simulink model "final_heart_sym3_2_Level_hdl"  (R2021a)
settings: Solver=VariableStepAuto  StartTime=0.0  StopTime=10.0  RelTol=1e-3
undefined symbols (not defined in the file or in its folder): lambda2
(part 1 of 2)
settings Model: Creator=Acer  LastModifiedBy=Acer

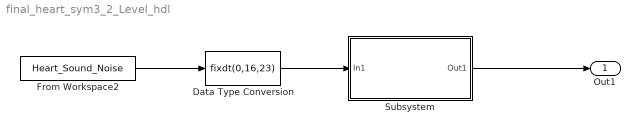
== system final_heart_sym3_2_Level_hdl ==
  Data Type Conversion : DataTypeConversion  OutDataTypeStr=fixdt(0,16,23)
  From Workspace2 : FromWorkspace  VariableName=Heart_Sound_Noise  OutDataTypeStr=double  SampleTime=1/44100
  Subsystem : Subsystem
  Out1 : Outport  OutDataTypeStr=fixdt(1,16,29)  SampleTime=1/44100
  wires:
  Subsystem/1(Out1) -> Out1/1
  From Workspace2/1 -> Data Type Conversion/1
  Data Type Conversion/1 -> Subsystem/1(In1)

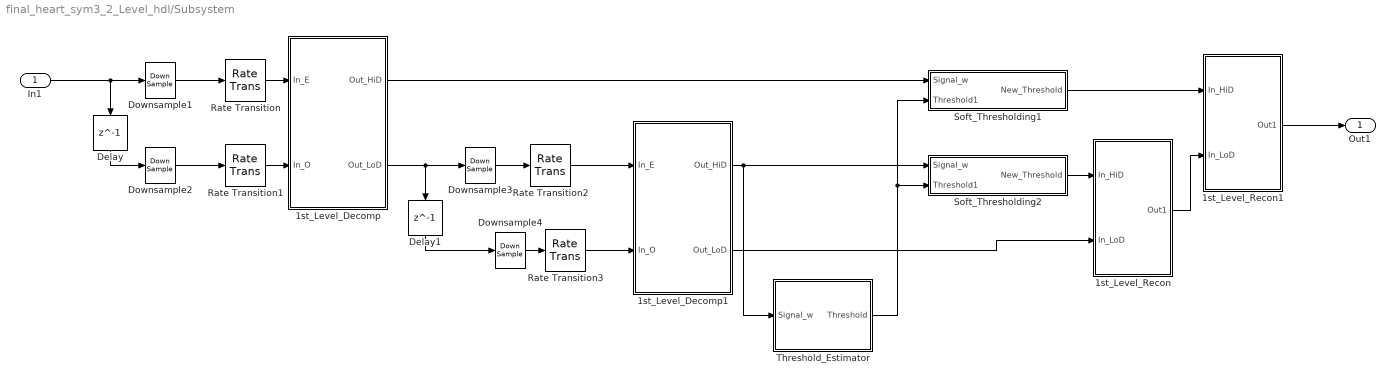
== system final_heart_sym3_2_Level_hdl/Subsystem ==
  In1 : Inport  OutDataTypeStr=fixdt(0,16,23)
  1st_Level_Decomp : Subsystem
  1st_Level_Decomp1 : Subsystem
  1st_Level_Recon : Subsystem
  1st_Level_Recon1 : Subsystem
  Delay : Delay  DelayLength=1  SampleTime=1/44100
  Delay1 : Delay  DelayLength=1  SampleTime=1/44100
  Downsample{1..4} (4 alike) : DownSample  N=30  RateOptions=Allow multirate processing
  Rate Transition{,1..3} (4 alike) : RateTransition
  Soft_Thresholding1 : Subsystem
  Soft_Thresholding2 : Subsystem
  Threshold_Estimator : Subsystem
  Out1 : Outport  OutDataTypeStr=fixdt(1,16,29)  SampleTime=1/44100
  wires:
  Rate Transition3/1 -> 1st_Level_Decomp1/2(In_O)
  Rate Transition1/1 -> 1st_Level_Decomp/2(In_O)
  1st_Level_Decomp1/1(Out_HiD) -> Threshold_Estimator/1(Signal_w), Soft_Thresholding2/1(Signal_w)
  Delay/1 -> Downsample2/1
  Soft_Thresholding1/1(New_Threshold) -> 1st_Level_Recon1/1(In_HiD)
  Downsample2/1 -> Rate Transition1/1
  1st_Level_Decomp/1(Out_HiD) -> Soft_Thresholding1/1(Signal_w)
  Delay1/1 -> Downsample4/1
  Downsample4/1 -> Rate Transition3/1
  1st_Level_Recon1/1(Out1) -> Out1/1
  Rate Transition2/1 -> 1st_Level_Decomp1/1(In_E)
  In1/1 -> Delay/1, Downsample1/1
  1st_Level_Decomp/2(Out_LoD) -> Downsample3/1, Delay1/1
  Soft_Thresholding2/1(New_Threshold) -> 1st_Level_Recon/1(In_HiD)
  Threshold_Estimator/1(Threshold) -> Soft_Thresholding2/2(Threshold1), Soft_Thresholding1/2(Threshold1)
  Downsample1/1 -> Rate Transition/1
  1st_Level_Recon/1(Out1) -> 1st_Level_Recon1/2(In_LoD)
  Rate Transition/1 -> 1st_Level_Decomp/1(In_E)
  Downsample3/1 -> Rate Transition2/1
  1st_Level_Decomp1/2(Out_LoD) -> 1st_Level_Recon/2(In_LoD)

== system final_heart_sym3_2_Level_hdl/Subsystem/1st_Level_Decomp ==
  In_E : Inport  OutDataTypeStr=fixdt(0,16,23)  SampleTime=1/44100
  In_O : Inport  Port=2  OutDataTypeStr=fixdt(0,16,23)  SampleTime=1/44100
  Add : Sum  AccumDataTypeStr=fixdt(1,16,23)  OutDataTypeStr=fixdt(1,16,24)
  Add1 : Sum  AccumDataTypeStr=fixdt(1,16,22)  OutDataTypeStr=fixdt(1,16,22)
  Delay1 : Delay  DelayLength=1  SampleTime=1/44100
  Delay2 : Delay  DelayLength=1  SampleTime=1/44100
  Gain : Gain  Gain=1/(0.877989329+0.977128821)  ParamDataTypeStr=fixdt(0,16,16)  OutDataTypeStr=fixdt(1,16,24)
  Gain1 : Gain  Gain=1/(0.877989329+0.977128821)  ParamDataTypeStr=fixdt(0,16,16)  OutDataTypeStr=fixdt(1,16,23)
  HiD_Even : Subsystem
  HiD_Odd : Subsystem
  LoD_Even : Subsystem
  LoD_Odd : Subsystem
  Out_HiD : Outport  OutDataTypeStr=fixdt(1,16,24)  SampleTime=1/44100  VectorParamsAs1DForOutWhenUnconnected=off
  Out_LoD : Outport  Port=2  OutDataTypeStr=fixdt(1,16,23)  SampleTime=1/44100  VectorParamsAs1DForOutWhenUnconnected=off
  wires:
  HiD_Odd/1(Out_HiD_o) -> Add/2
  HiD_Even/1(Out_HiD_e) -> Add/1
  LoD_Odd/1(Out_LoD_o) -> Add1/2
  LoD_Even/1(Out_LoD_e) -> Add1/1
  In_E/1 -> LoD_Even/1(In_LoD_e), HiD_Even/1(In_HiD_e)
  In_O/1 -> LoD_Odd/1(In_LoD_o), HiD_Odd/1(In_HiD_o)
  Gain/1 -> Delay1/1
  Delay1/1 -> Out_HiD/1
  Delay2/1 -> Out_LoD/1
  Add/1 -> Gain/1
  Add1/1 -> Gain1/1
  Gain1/1 -> Delay2/1

== system final_heart_sym3_2_Level_hdl/Subsystem/1st_Level_Decomp1 ==
  In_E : Inport  OutDataTypeStr=fixdt(1,16,4)  SampleTime=1/44100
  In_O : Inport  Port=2  OutDataTypeStr=fixdt(1,16,4)  SampleTime=1/44100
  Add : Sum  AccumDataTypeStr=fixdt(1,16,4)  OutDataTypeStr=fixdt(1,16,4)
  Add1 : Sum  AccumDataTypeStr=fixdt(1,16,4)  OutDataTypeStr=fixdt(1,16,4)
  Delay1 : Delay  DelayLength=1  SampleTime=1/44100
  Delay2 : Delay  DelayLength=1  SampleTime=1/44100
  Gain : Gain  Gain=1/(0.877989329+0.977128821)  ParamDataTypeStr=fixdt(0,16,16)  OutDataTypeStr=fixdt(1,16,4)
  Gain1 : Gain  Gain=1/(0.877989329+0.977128821)  ParamDataTypeStr=fixdt(0,16,16)  OutDataTypeStr=fixdt(1,16,4)
  HiD_Even : Subsystem
  HiD_Odd : Subsystem
  LoD_Even : Subsystem
  LoD_Odd : Subsystem
  Out_HiD : Outport  OutDataTypeStr=fixdt(1,16,4)  SampleTime=1/44100  VectorParamsAs1DForOutWhenUnconnected=off
  Out_LoD : Outport  Port=2  OutDataTypeStr=fixdt(1,16,4)  SampleTime=1/44100  VectorParamsAs1DForOutWhenUnconnected=off
  wires:
  HiD_Odd/1(Out_HiD_o) -> Add/2
  HiD_Even/1(Out_HiD_e) -> Add/1
  LoD_Odd/1(Out_LoD_o) -> Add1/2
  LoD_Even/1(Out_LoD_e) -> Add1/1
  In_E/1 -> LoD_Even/1(In_LoD_e), HiD_Even/1(In_HiD_e)
  In_O/1 -> LoD_Odd/1(In_LoD_o), HiD_Odd/1(In_HiD_o)
  Gain/1 -> Delay1/1
  Delay1/1 -> Out_HiD/1
  Delay2/1 -> Out_LoD/1
  Add/1 -> Gain/1
  Add1/1 -> Gain1/1
  Gain1/1 -> Delay2/1

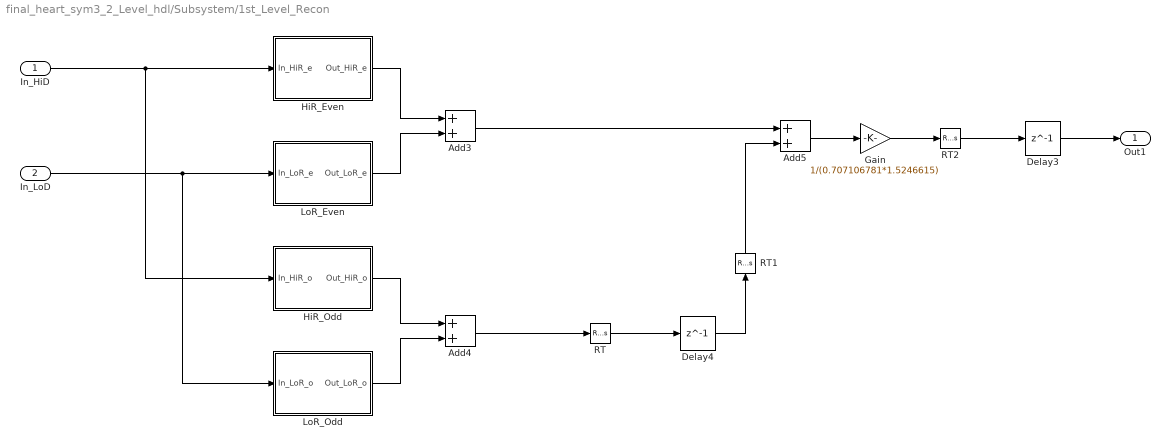
== system final_heart_sym3_2_Level_hdl/Subsystem/1st_Level_Recon ==
  In_HiD : Inport  OutDataTypeStr=fixdt(1,16,4)  SampleTime=1/44100
  In_LoD : Inport  Port=2  OutDataTypeStr=fixdt(1,16,4)  SampleTime=1/44100
  Add3 : Sum  AccumDataTypeStr=fixdt(1,16,4)  OutDataTypeStr=fixdt(1,16,4)
  Add4 : Sum  AccumDataTypeStr=fixdt(1,16,4)  OutDataTypeStr=fixdt(1,16,4)
  Add5 : Sum  AccumDataTypeStr=fixdt(1,16,4)  OutDataTypeStr=fixdt(1,16,4)
  Delay3 : Delay  DelayLength=1  SampleTime=1/44100
  Delay4 : Delay  DelayLength=1  SampleTime=1/44100
  Gain : Gain  Gain=1/(0.707106781*1.5246615)  ParamDataTypeStr=fixdt(0,16,16)  OutDataTypeStr=fixdt(1,16,4)
  HiR_Even : Subsystem
  HiR_Odd : Subsystem
  LoR_Even : Subsystem
  LoR_Odd : Subsystem
  RT : RateTransition
  RT1 : RateTransition
  RT2 : RateTransition
  Out1 : Outport  OutDataTypeStr=fixdt(1,16,4)  SampleTime=1/44100
  wires:
  In_HiD/1 -> HiR_Odd/1(In_HiR_o), HiR_Even/1(In_HiR_e)
  HiR_Even/1(Out_HiR_e) -> Add3/1
  In_LoD/1 -> LoR_Odd/1(In_LoR_o), LoR_Even/1(In_LoR_e)
  LoR_Even/1(Out_LoR_e) -> Add3/2
  HiR_Odd/1(Out_HiR_o) -> Add4/1
  LoR_Odd/1(Out_LoR_o) -> Add4/2
  RT/1 -> Delay4/1
  Delay3/1 -> Out1/1
  RT1/1 -> Add5/2
  RT2/1 -> Delay3/1
  Delay4/1 -> RT1/1
  Add5/1 -> Gain/1
  Gain/1 -> RT2/1
  Add3/1 -> Add5/1
  Add4/1 -> RT/1

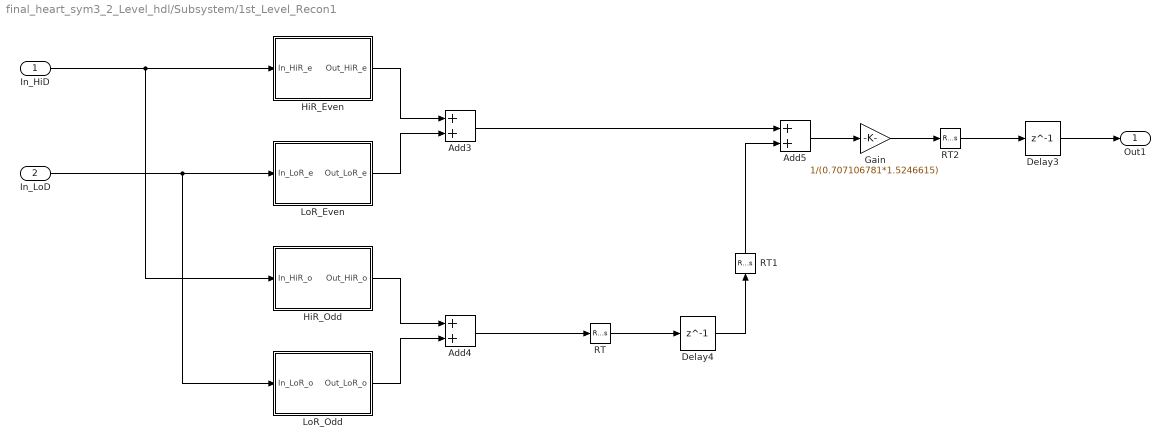
== system final_heart_sym3_2_Level_hdl/Subsystem/1st_Level_Recon1 ==
  In_HiD : Inport  OutDataTypeStr=fixdt(1,16,28)  SampleTime=1/44100
  In_LoD : Inport  Port=2  OutDataTypeStr=fixdt(1,16,4)  SampleTime=1/44100
  Add3 : Sum  AccumDataTypeStr=fixdt(1,16,28)  OutDataTypeStr=fixdt(1,16,28)
  Add4 : Sum  AccumDataTypeStr=fixdt(1,16,28)  OutDataTypeStr=fixdt(1,16,28)
  Add5 : Sum  AccumDataTypeStr=fixdt(1,16,28)  OutDataTypeStr=fixdt(1,16,29)
  Delay3 : Delay  DelayLength=1  SampleTime=1/44100
  Delay4 : Delay  DelayLength=1  SampleTime=1/44100
  Gain : Gain  Gain=1/(0.707106781*1.5246615)  ParamDataTypeStr=fixdt(0,16,16)  OutDataTypeStr=fixdt(1,16,29)
  HiR_Even : Subsystem
  HiR_Odd : Subsystem
  LoR_Even : Subsystem
  LoR_Odd : Subsystem
  RT : RateTransition
  RT1 : RateTransition
  RT2 : RateTransition
  Out1 : Outport  OutDataTypeStr=fixdt(1,16,29)  SampleTime=1/44100
  wires:
  In_HiD/1 -> HiR_Odd/1(In_HiR_o), HiR_Even/1(In_HiR_e)
  HiR_Even/1(Out_HiR_e) -> Add3/1
  In_LoD/1 -> LoR_Odd/1(In_LoR_o), LoR_Even/1(In_LoR_e)
  LoR_Even/1(Out_LoR_e) -> Add3/2
  HiR_Odd/1(Out_HiR_o) -> Add4/1
  LoR_Odd/1(Out_LoR_o) -> Add4/2
  RT/1 -> Delay4/1
  Delay3/1 -> Out1/1
  RT1/1 -> Add5/2
  RT2/1 -> Delay3/1
  Delay4/1 -> RT1/1
  Add5/1 -> Gain/1
  Gain/1 -> RT2/1
  Add3/1 -> Add5/1
  Add4/1 -> RT/1

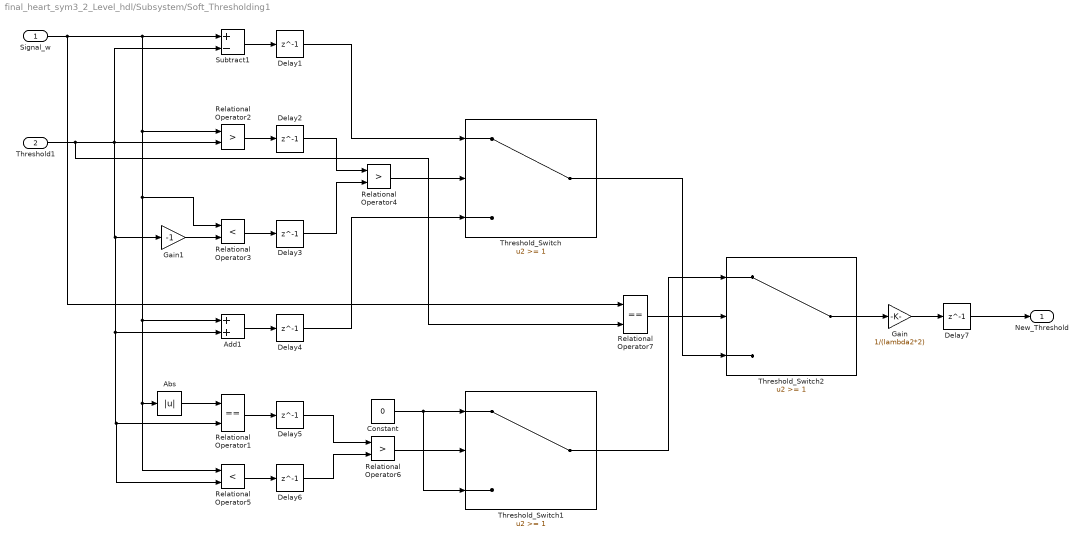
== system final_heart_sym3_2_Level_hdl/Subsystem/Soft_Thresholding1 ==
  Signal_w : Inport  OutDataTypeStr=fixdt(1,16,24)  SampleTime=1/44100
  Threshold1 : Inport  Port=2  OutDataTypeStr=fixdt(1,16,4)  SampleTime=1/44100
  Abs : Abs  OutDataTypeStr=fixdt(0,16,25)
  Add1 : Sum  AccumDataTypeStr=fixdt(1,16,24)  OutDataTypeStr=fixdt(1,16,24)
  Constant : Constant  Value=0  OutDataTypeStr=fixdt(1,16,4)  SampleTime=1/44100
  Delay{1..7} (7 alike) : Delay  DelayLength=1  SampleTime=1/44100
  Gain : Gain  Gain=1/(lambda2*2)  ParamDataTypeStr=fixdt(0,16,19)  OutDataTypeStr=fixdt(1,16,28)
  Gain1 : Gain  Gain=-1  ParamDataTypeStr=fixdt(1,16,15)  OutMin=-1  OutMax=-0.99  OutDataTypeStr=fixdt(1,16,15)
  Relational Operator1 : RelationalOperator  Operator===  OutDataTypeStr=boolean  RndMeth=Simplest
  Relational Operator2 : RelationalOperator  Operator=>  OutDataTypeStr=boolean  RndMeth=Simplest
  Relational Operator3 : RelationalOperator  Operator=<  OutDataTypeStr=boolean  RndMeth=Simplest
  Relational Operator4 : RelationalOperator  Operator=>  OutDataTypeStr=boolean  RndMeth=Simplest
  Relational Operator5 : RelationalOperator  Operator=<  OutDataTypeStr=boolean  RndMeth=Simplest
  Relational Operator6 : RelationalOperator  Operator=>  OutDataTypeStr=boolean  RndMeth=Simplest
  Relational Operator7 : RelationalOperator  Operator===  OutDataTypeStr=boolean  RndMeth=Simplest
  Subtract1 : Sum  Inputs=+-  AccumDataTypeStr=fixdt(1,16,24)  OutDataTypeStr=fixdt(1,16,24)
  Threshold_Switch : Switch  Threshold=1  OutDataTypeStr=fixdt(1,16,24)
  Threshold_Switch1 : Switch  Threshold=1  OutDataTypeStr=fixdt(1,16,4)
  Threshold_Switch2 : Switch  Threshold=1  OutDataTypeStr=fixdt(1,16,24)
  New_Threshold : Outport  OutDataTypeStr=fixdt(1,16,28)  SampleTime=1/44100
  wires:
  Threshold_Switch/1 -> Threshold_Switch2/3
  Relational Operator6/1 -> Threshold_Switch1/2
  Gain1/1 -> Relational Operator3/2
  Delay4/1 -> Threshold_Switch/3
  Add1/1 -> Delay4/1
  Delay2/1 -> Relational Operator4/1
  Delay3/1 -> Relational Operator4/2
  Delay1/1 -> Threshold_Switch/1
  Relational Operator2/1 -> Delay2/1
  Relational Operator3/1 -> Delay3/1
  Relational Operator5/1 -> Delay6/1
  Delay6/1 -> Relational Operator6/2
  Delay5/1 -> Relational Operator6/1
  Threshold1/1 -> Relational Operator2/2, Subtract1/2, Relational Operator5/2, Relational Operator1/2, Add1/2, Gain1/1, Relational Operator7/2
  Abs/1 -> Relational Operator1/1
  Relational Operator4/1 -> Threshold_Switch/2
  Subtract1/1 -> Delay1/1
  Constant/1 -> Threshold_Switch1/3, Threshold_Switch1/1
  Signal_w/1 -> Subtract1/1, Relational Operator2/1, Relational Operator5/1, Abs/1, Add1/1, Relational Operator3/1, Relational Operator7/1
  Relational Operator7/1 -> Threshold_Switch2/2
  Relational Operator1/1 -> Delay5/1
  Threshold_Switch1/1 -> Threshold_Switch2/1
  Delay7/1 -> New_Threshold/1
  Threshold_Switch2/1 -> Gain/1
  Gain/1 -> Delay7/1

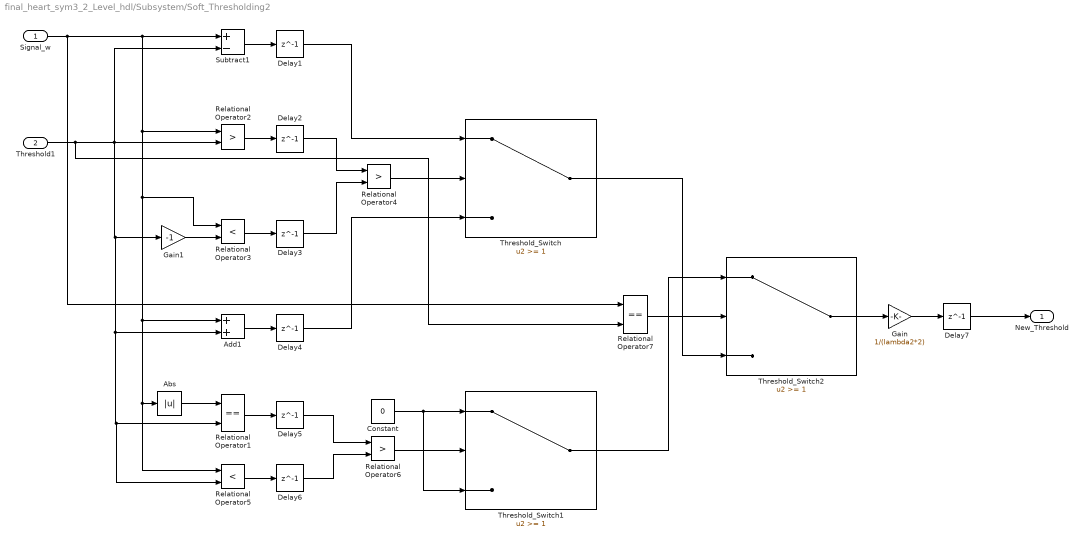
== system final_heart_sym3_2_Level_hdl/Subsystem/Soft_Thresholding2 ==
  Signal_w : Inport  OutDataTypeStr=fixdt(1,16,4)  SampleTime=1/44100
  Threshold1 : Inport  Port=2  OutDataTypeStr=fixdt(1,16,4)  SampleTime=1/44100
  Abs : Abs  OutDataTypeStr=fixdt(1,16,4)
  Add1 : Sum  AccumDataTypeStr=fixdt(1,16,4)  OutDataTypeStr=fixdt(1,16,4)
  Constant : Constant  Value=0  OutDataTypeStr=fixdt(1,16,4)  SampleTime=1/44100
  Delay{1..7} (7 alike) : Delay  DelayLength=1  SampleTime=1/44100
  Gain : Gain  Gain=1/(lambda2*2)  ParamDataTypeStr=fixdt(0,16,19)  OutDataTypeStr=fixdt(1,16,4)
  Gain1 : Gain  Gain=-1  ParamDataTypeStr=fixdt(1,16,15)  OutMin=-1  OutMax=-0.99  OutDataTypeStr=fixdt(1,16,15)
  Relational Operator1 : RelationalOperator  Operator===  OutDataTypeStr=boolean  RndMeth=Simplest
  Relational Operator2 : RelationalOperator  Operator=>  OutDataTypeStr=boolean  RndMeth=Simplest
  Relational Operator3 : RelationalOperator  Operator=<  OutDataTypeStr=boolean  RndMeth=Simplest
  Relational Operator4 : RelationalOperator  Operator=>  OutDataTypeStr=boolean  RndMeth=Simplest
  Relational Operator5 : RelationalOperator  Operator=<  OutDataTypeStr=boolean  RndMeth=Simplest
  Relational Operator6 : RelationalOperator  Operator=>  OutDataTypeStr=boolean  RndMeth=Simplest
  Relational Operator7 : RelationalOperator  Operator===  OutDataTypeStr=boolean  RndMeth=Simplest
  Subtract1 : Sum  Inputs=+-  AccumDataTypeStr=fixdt(1,16,4)  OutDataTypeStr=fixdt(1,16,4)
  Threshold_Switch : Switch  Threshold=1  OutDataTypeStr=fixdt(1,16,4)
  Threshold_Switch1 : Switch  Threshold=1  OutDataTypeStr=fixdt(1,16,4)
  Threshold_Switch2 : Switch  Threshold=1  OutDataTypeStr=fixdt(1,16,4)
  New_Threshold : Outport  OutDataTypeStr=fixdt(1,16,4)  SampleTime=1/44100
  wires:
  Threshold_Switch/1 -> Threshold_Switch2/3
  Relational Operator6/1 -> Threshold_Switch1/2
  Gain1/1 -> Relational Operator3/2
  Delay4/1 -> Threshold_Switch/3
  Add1/1 -> Delay4/1
  Delay2/1 -> Relational Operator4/1
  Delay3/1 -> Relational Operator4/2
  Delay1/1 -> Threshold_Switch/1
  Relational Operator2/1 -> Delay2/1
  Relational Operator3/1 -> Delay3/1
  Relational Operator5/1 -> Delay6/1
  Delay6/1 -> Relational Operator6/2
  Delay5/1 -> Relational Operator6/1
  Threshold1/1 -> Relational Operator2/2, Subtract1/2, Relational Operator5/2, Relational Operator1/2, Add1/2, Gain1/1, Relational Operator7/2
  Abs/1 -> Relational Operator1/1
  Relational Operator4/1 -> Threshold_Switch/2
  Subtract1/1 -> Delay1/1
  Constant/1 -> Threshold_Switch1/3, Threshold_Switch1/1
  Signal_w/1 -> Subtract1/1, Relational Operator2/1, Relational Operator5/1, Abs/1, Add1/1, Relational Operator3/1, Relational Operator7/1
  Relational Operator7/1 -> Threshold_Switch2/2
  Relational Operator1/1 -> Delay5/1
  Threshold_Switch1/1 -> Threshold_Switch2/1
  Delay7/1 -> New_Threshold/1
  Threshold_Switch2/1 -> Gain/1
  Gain/1 -> Delay7/1

== system final_heart_sym3_2_Level_hdl/Subsystem/Threshold_Estimator ==
  Signal_w : Inport  OutDataTypeStr=fixdt(1,16,4)  SampleTime=1/44100
  Absolute_Value1 : Subsystem
  Length : Constant  Value=lambda2  OutDataTypeStr=fixdt(0,16,13)  SampleTime=1/44100
  Median2 : Subsystem
  Multiply : Product  OutDataTypeStr=fixdt(1,16,4)
  Threshold : Outport  OutDataTypeStr=fixdt(1,16,4)  SampleTime=1/44100  VectorParamsAs1DForOutWhenUnconnected=off
  wires:
  Length/1 -> Multiply/2
  Median2/1(Median) -> Multiply/1
  Absolute_Value1/1(Out_Abs) -> Median2/1(Signal_w3)
  Signal_w/1 -> Absolute_Value1/1(Signal_w4)
  Multiply/1 -> Threshold/1

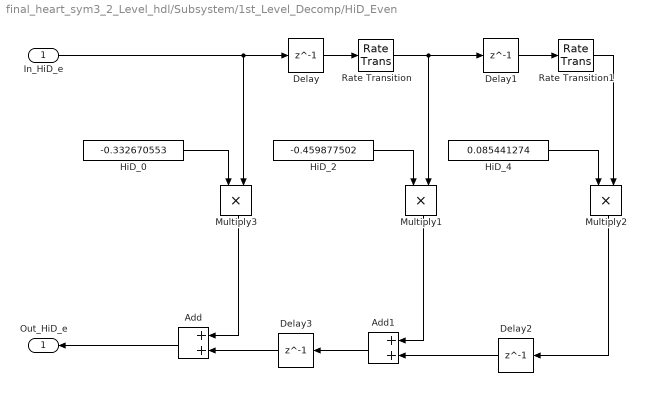
== system final_heart_sym3_2_Level_hdl/Subsystem/1st_Level_Decomp/HiD_Even ==
  In_HiD_e : Inport  OutDataTypeStr=fixdt(0,16,23)  SampleTime=1/44100
  Add : Sum  AccumDataTypeStr=fixdt(1,16,23)  OutDataTypeStr=fixdt(1,16,23)
  Add1 : Sum  AccumDataTypeStr=fixdt(1,16,23)  OutDataTypeStr=fixdt(1,16,24)
  Delay{,1..3} (4 alike) : Delay  DelayLength=1  SampleTime=1/44100
  HiD_0 : Constant  Value=-0.332670553  OutDataTypeStr=fixdt(1,16,16)  SampleTime=1/44100
  HiD_2 : Constant  Value=-0.459877502  OutDataTypeStr=fixdt(1,16,16)  SampleTime=1/44100
  HiD_4 : Constant  Value=0.085441274  OutDataTypeStr=fixdt(0,16,19)  SampleTime=1/44100
  Multiply1 : Product  OutDataTypeStr=fixdt(1,16,15)
  Multiply2 : Product  OutDataTypeStr=fixdt(0,16,27)
  Multiply3 : Product  OutDataTypeStr=fixdt(1,16,15)
  Rate Transition : RateTransition
  Rate Transition1 : RateTransition
  Out_HiD_e : Outport  OutDataTypeStr=fixdt(1,16,23)  SampleTime=1/44100  VectorParamsAs1DForOutWhenUnconnected=off
  wires:
  In_HiD_e/1 -> Multiply3/2, Delay/1
  Multiply3/1 -> Add/1
  HiD_0/1 -> Multiply3/1
  HiD_2/1 -> Multiply1/1
  Add/1 -> Out_HiD_e/1
  Multiply2/1 -> Delay2/1
  Multiply1/1 -> Add1/1
  Delay2/1 -> Add1/2
  Add1/1 -> Delay3/1
  Delay3/1 -> Add/2
  HiD_4/1 -> Multiply2/1
  Rate Transition1/1 -> Multiply2/2
  Delay1/1 -> Rate Transition1/1
  Rate Transition/1 -> Multiply1/2, Delay1/1
  Delay/1 -> Rate Transition/1

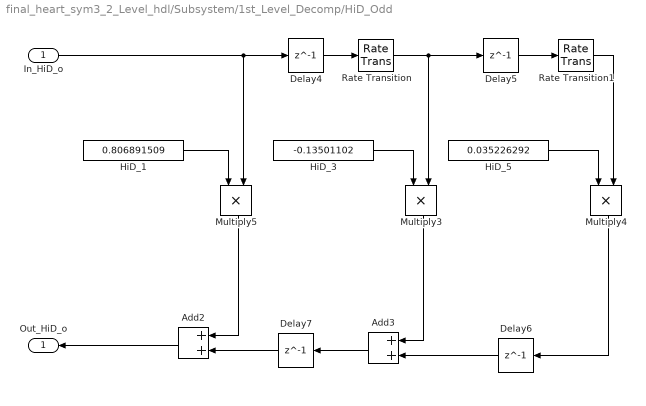
== system final_heart_sym3_2_Level_hdl/Subsystem/1st_Level_Decomp/HiD_Odd ==
  In_HiD_o : Inport  OutDataTypeStr=fixdt(0,16,23)  SampleTime=1/44100
  Add2 : Sum  AccumDataTypeStr=fixdt(1,16,23)  OutDataTypeStr=fixdt(1,16,23)
  Add3 : Sum  AccumDataTypeStr=fixdt(1,16,25)  OutDataTypeStr=fixdt(1,16,25)
  Delay{4..7} (4 alike) : Delay  DelayLength=1  SampleTime=1/44100
  HiD_1 : Constant  Value=0.806891509  OutDataTypeStr=fixdt(0,16,16)  SampleTime=1/44100
  HiD_3 : Constant  Value=-0.13501102  OutDataTypeStr=fixdt(1,16,17)  SampleTime=1/44100
  HiD_5 : Constant  Value=0.035226292  OutDataTypeStr=fixdt(0,16,20)  SampleTime=1/44100
  Multiply3 : Product  OutDataTypeStr=fixdt(1,16,15)
  Multiply4 : Product  OutDataTypeStr=fixdt(0,16,28)
  Multiply5 : Product  OutDataTypeStr=fixdt(0,16,24)
  Rate Transition : RateTransition
  Rate Transition1 : RateTransition
  Out_HiD_o : Outport  OutDataTypeStr=fixdt(1,16,23)  SampleTime=1/44100  VectorParamsAs1DForOutWhenUnconnected=off
  wires:
  Delay5/1 -> Rate Transition1/1
  Rate Transition1/1 -> Multiply4/2
  HiD_3/1 -> Multiply3/1
  Add3/1 -> Delay7/1
  Delay7/1 -> Add2/2
  HiD_5/1 -> Multiply4/1
  In_HiD_o/1 -> Multiply5/2, Delay4/1
  Multiply5/1 -> Add2/1
  Add2/1 -> Out_HiD_o/1
  Multiply4/1 -> Delay6/1
  Multiply3/1 -> Add3/1
  Delay4/1 -> Rate Transition/1
  HiD_1/1 -> Multiply5/1
  Delay6/1 -> Add3/2
  Rate Transition/1 -> Multiply3/2, Delay5/1

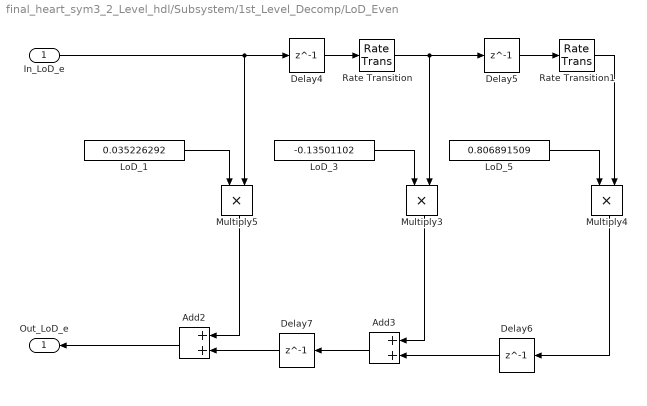
== system final_heart_sym3_2_Level_hdl/Subsystem/1st_Level_Decomp/LoD_Even ==
  In_LoD_e : Inport  OutDataTypeStr=fixdt(0,16,23)  SampleTime=1/44100
  Add2 : Sum  AccumDataTypeStr=fixdt(1,16,23)  OutDataTypeStr=fixdt(1,16,23)
  Add3 : Sum  AccumDataTypeStr=fixdt(1,16,23)  OutDataTypeStr=fixdt(1,16,23)
  Delay{4..7} (4 alike) : Delay  DelayLength=1  SampleTime=1/44100
  LoD_1 : Constant  Value=0.035226292  OutDataTypeStr=fixdt(0,16,20)  SampleTime=1/44100
  LoD_3 : Constant  Value=-0.13501102  OutDataTypeStr=fixdt(1,16,17)  SampleTime=1/44100
  LoD_5 : Constant  Value=0.806891509  OutDataTypeStr=fixdt(0,16,16)  SampleTime=1/44100
  Multiply3 : Product  OutDataTypeStr=fixdt(1,16,15)
  Multiply4 : Product  OutDataTypeStr=fixdt(0,16,24)
  Multiply5 : Product  OutDataTypeStr=fixdt(0,16,28)
  Rate Transition : RateTransition
  Rate Transition1 : RateTransition
  Out_LoD_e : Outport  OutDataTypeStr=fixdt(1,16,23)  SampleTime=1/44100  VectorParamsAs1DForOutWhenUnconnected=off
  wires:
  Delay5/1 -> Rate Transition1/1
  Rate Transition1/1 -> Multiply4/2
  LoD_3/1 -> Multiply3/1
  Add3/1 -> Delay7/1
  Delay7/1 -> Add2/2
  LoD_5/1 -> Multiply4/1
  In_LoD_e/1 -> Multiply5/2, Delay4/1
  Multiply5/1 -> Add2/1
  Add2/1 -> Out_LoD_e/1
  Multiply4/1 -> Delay6/1
  Multiply3/1 -> Add3/1
  Delay4/1 -> Rate Transition/1
  LoD_1/1 -> Multiply5/1
  Delay6/1 -> Add3/2
  Rate Transition/1 -> Multiply3/2, Delay5/1

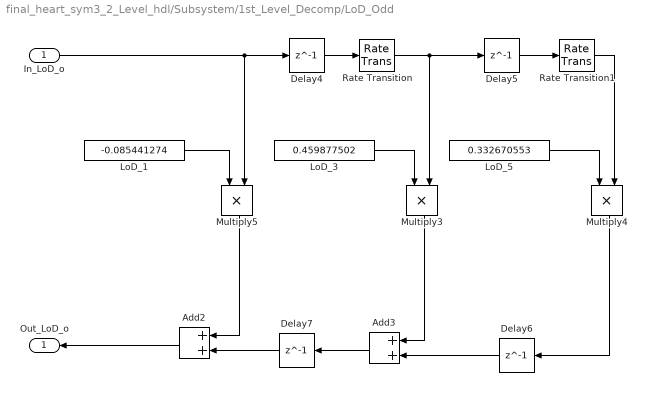
== system final_heart_sym3_2_Level_hdl/Subsystem/1st_Level_Decomp/LoD_Odd ==
  In_LoD_o : Inport  OutDataTypeStr=fixdt(0,16,23)  SampleTime=1/44100
  Add2 : Sum  AccumDataTypeStr=fixdt(1,16,23)  OutDataTypeStr=fixdt(1,16,23)
  Add3 : Sum  AccumDataTypeStr=fixdt(0,16,24)  OutDataTypeStr=fixdt(0,16,24)
  Delay{4..7} (4 alike) : Delay  DelayLength=1  SampleTime=1/44100
  LoD_1 : Constant  Value=-0.085441274  OutDataTypeStr=fixdt(1,16,18)  SampleTime=1/44100
  LoD_3 : Constant  Value=0.459877502  OutDataTypeStr=fixdt(0,16,17)  SampleTime=1/44100
  LoD_5 : Constant  Value=0.332670553  OutDataTypeStr=fixdt(0,16,17)  SampleTime=1/44100
  Multiply3 : Product  OutDataTypeStr=fixdt(0,16,24)
  Multiply4 : Product  OutDataTypeStr=fixdt(0,16,25)
  Multiply5 : Product  OutDataTypeStr=fixdt(1,16,15)
  Rate Transition : RateTransition
  Rate Transition1 : RateTransition
  Out_LoD_o : Outport  OutDataTypeStr=fixdt(1,16,23)  SampleTime=1/44100  VectorParamsAs1DForOutWhenUnconnected=off
  wires:
  Delay5/1 -> Rate Transition1/1
  Rate Transition1/1 -> Multiply4/2
  LoD_3/1 -> Multiply3/1
  Add3/1 -> Delay7/1
  Delay7/1 -> Add2/2
  LoD_5/1 -> Multiply4/1
  In_LoD_o/1 -> Multiply5/2, Delay4/1
  Multiply5/1 -> Add2/1
  Add2/1 -> Out_LoD_o/1
  Multiply4/1 -> Delay6/1
  Multiply3/1 -> Add3/1
  Delay4/1 -> Rate Transition/1
  LoD_1/1 -> Multiply5/1
  Delay6/1 -> Add3/2
  Rate Transition/1 -> Multiply3/2, Delay5/1

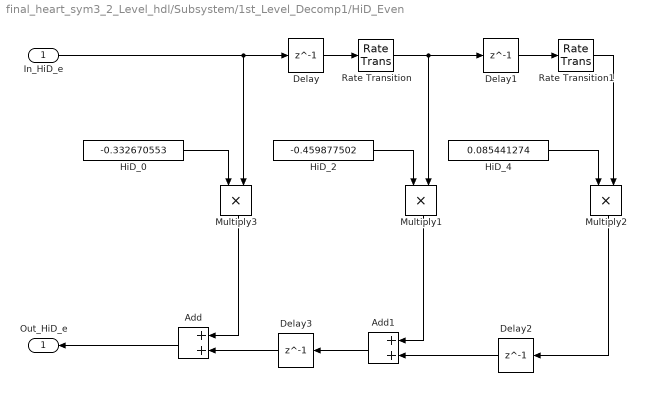
== system final_heart_sym3_2_Level_hdl/Subsystem/1st_Level_Decomp1/HiD_Even ==
  In_HiD_e : Inport  OutDataTypeStr=fixdt(1,16,4)  SampleTime=1/44100
  Add : Sum  AccumDataTypeStr=fixdt(1,16,4)  OutDataTypeStr=fixdt(1,16,4)
  Add1 : Sum  AccumDataTypeStr=fixdt(1,16,4)  OutDataTypeStr=fixdt(1,16,4)
  Delay{,1..3} (4 alike) : Delay  DelayLength=1  SampleTime=1/44100
  HiD_0 : Constant  Value=-0.332670553  OutDataTypeStr=fixdt(1,16,16)  SampleTime=1/44100
  HiD_2 : Constant  Value=-0.459877502  OutDataTypeStr=fixdt(1,16,16)  SampleTime=1/44100
  HiD_4 : Constant  Value=0.085441274  OutDataTypeStr=fixdt(0,16,19)  SampleTime=1/44100
  Multiply1 : Product  OutDataTypeStr=fixdt(1,16,4)
  Multiply2 : Product  OutDataTypeStr=fixdt(1,16,4)
  Multiply3 : Product  OutDataTypeStr=fixdt(1,16,4)
  Rate Transition : RateTransition
  Rate Transition1 : RateTransition
  Out_HiD_e : Outport  OutDataTypeStr=fixdt(1,16,4)  SampleTime=1/44100  VectorParamsAs1DForOutWhenUnconnected=off
  wires:
  In_HiD_e/1 -> Multiply3/2, Delay/1
  Multiply3/1 -> Add/1
  HiD_0/1 -> Multiply3/1
  HiD_2/1 -> Multiply1/1
  Add/1 -> Out_HiD_e/1
  Multiply2/1 -> Delay2/1
  Multiply1/1 -> Add1/1
  Delay2/1 -> Add1/2
  Add1/1 -> Delay3/1
  Delay3/1 -> Add/2
  HiD_4/1 -> Multiply2/1
  Rate Transition1/1 -> Multiply2/2
  Delay1/1 -> Rate Transition1/1
  Rate Transition/1 -> Multiply1/2, Delay1/1
  Delay/1 -> Rate Transition/1

== system final_heart_sym3_2_Level_hdl/Subsystem/1st_Level_Decomp1/HiD_Odd ==
  In_HiD_o : Inport  OutDataTypeStr=fixdt(1,16,4)  SampleTime=1/44100
  Add2 : Sum  AccumDataTypeStr=fixdt(1,16,4)  OutDataTypeStr=fixdt(1,16,4)
  Add3 : Sum  AccumDataTypeStr=fixdt(1,16,4)  OutDataTypeStr=fixdt(1,16,4)
  Delay{4..7} (4 alike) : Delay  DelayLength=1  SampleTime=1/44100
  HiD_1 : Constant  Value=0.806891509  OutDataTypeStr=fixdt(0,16,16)  SampleTime=1/44100
  HiD_3 : Constant  Value=-0.13501102  OutDataTypeStr=fixdt(1,16,17)  SampleTime=1/44100
  HiD_5 : Constant  Value=0.035226292  OutDataTypeStr=fixdt(0,16,20)  SampleTime=1/44100
  Multiply3 : Product  OutDataTypeStr=fixdt(1,16,4)
  Multiply4 : Product  OutDataTypeStr=fixdt(1,16,4)
  Multiply5 : Product  OutDataTypeStr=fixdt(1,16,4)
  Rate Transition : RateTransition
  Rate Transition1 : RateTransition
  Out_HiD_o : Outport  OutDataTypeStr=fixdt(1,16,4)  SampleTime=1/44100  VectorParamsAs1DForOutWhenUnconnected=off
  wires:
  Delay5/1 -> Rate Transition1/1
  Rate Transition1/1 -> Multiply4/2
  HiD_3/1 -> Multiply3/1
  Add3/1 -> Delay7/1
  Delay7/1 -> Add2/2
  HiD_5/1 -> Multiply4/1
  In_HiD_o/1 -> Multiply5/2, Delay4/1
  Multiply5/1 -> Add2/1
  Add2/1 -> Out_HiD_o/1
  Multiply4/1 -> Delay6/1
  Multiply3/1 -> Add3/1
  Delay4/1 -> Rate Transition/1
  HiD_1/1 -> Multiply5/1
  Delay6/1 -> Add3/2
  Rate Transition/1 -> Multiply3/2, Delay5/1

== system final_heart_sym3_2_Level_hdl/Subsystem/1st_Level_Decomp1/LoD_Even ==
  In_LoD_e : Inport  OutDataTypeStr=fixdt(1,16,4)  SampleTime=1/44100
  Add2 : Sum  AccumDataTypeStr=fixdt(1,16,4)  OutDataTypeStr=fixdt(1,16,4)
  Add3 : Sum  AccumDataTypeStr=fixdt(1,16,4)  OutDataTypeStr=fixdt(1,16,4)
  Delay{4..7} (4 alike) : Delay  DelayLength=1  SampleTime=1/44100
  LoD_1 : Constant  Value=0.035226292  OutDataTypeStr=fixdt(0,16,20)  SampleTime=1/44100
  LoD_3 : Constant  Value=-0.13501102  OutDataTypeStr=fixdt(1,16,17)  SampleTime=1/44100
  LoD_5 : Constant  Value=0.806891509  OutDataTypeStr=fixdt(0,16,16)  SampleTime=1/44100
  Multiply3 : Product  OutDataTypeStr=fixdt(1,16,4)
  Multiply4 : Product  OutDataTypeStr=fixdt(1,16,4)
  Multiply5 : Product  OutDataTypeStr=fixdt(1,16,4)
  Rate Transition : RateTransition
  Rate Transition1 : RateTransition
  Out_LoD_e : Outport  OutDataTypeStr=fixdt(1,16,4)  SampleTime=1/44100  VectorParamsAs1DForOutWhenUnconnected=off
  wires:
  Delay5/1 -> Rate Transition1/1
  Rate Transition1/1 -> Multiply4/2
  LoD_3/1 -> Multiply3/1
  Add3/1 -> Delay7/1
  Delay7/1 -> Add2/2
  LoD_5/1 -> Multiply4/1
  In_LoD_e/1 -> Multiply5/2, Delay4/1
  Multiply5/1 -> Add2/1
  Add2/1 -> Out_LoD_e/1
  Multiply4/1 -> Delay6/1
  Multiply3/1 -> Add3/1
  Delay4/1 -> Rate Transition/1
  LoD_1/1 -> Multiply5/1
  Delay6/1 -> Add3/2
  Rate Transition/1 -> Multiply3/2, Delay5/1

== system final_heart_sym3_2_Level_hdl/Subsystem/1st_Level_Decomp1/LoD_Odd ==
  In_LoD_o : Inport  OutDataTypeStr=fixdt(1,16,4)  SampleTime=1/44100
  Add2 : Sum  AccumDataTypeStr=fixdt(1,16,4)  OutDataTypeStr=fixdt(1,16,4)
  Add3 : Sum  AccumDataTypeStr=fixdt(1,16,4)  OutDataTypeStr=fixdt(1,16,4)
  Delay{4..7} (4 alike) : Delay  DelayLength=1  SampleTime=1/44100
  LoD_1 : Constant  Value=-0.085441274  OutDataTypeStr=fixdt(1,16,18)  SampleTime=1/44100
  LoD_3 : Constant  Value=0.459877502  OutDataTypeStr=fixdt(0,16,17)  SampleTime=1/44100
  LoD_5 : Constant  Value=0.332670553  OutDataTypeStr=fixdt(0,16,17)  SampleTime=1/44100
  Multiply3 : Product  OutDataTypeStr=fixdt(1,16,4)
  Multiply4 : Product  OutDataTypeStr=fixdt(1,16,4)
  Multiply5 : Product  OutDataTypeStr=fixdt(1,16,4)
  Rate Transition : RateTransition
  Rate Transition1 : RateTransition
  Out_LoD_o : Outport  OutDataTypeStr=fixdt(1,16,4)  SampleTime=1/44100  VectorParamsAs1DForOutWhenUnconnected=off
  wires:
  Delay5/1 -> Rate Transition1/1
  Rate Transition1/1 -> Multiply4/2
  LoD_3/1 -> Multiply3/1
  Add3/1 -> Delay7/1
  Delay7/1 -> Add2/2
  LoD_5/1 -> Multiply4/1
  In_LoD_o/1 -> Multiply5/2, Delay4/1
  Multiply5/1 -> Add2/1
  Add2/1 -> Out_LoD_o/1
  Multiply4/1 -> Delay6/1
  Multiply3/1 -> Add3/1
  Delay4/1 -> Rate Transition/1
  LoD_1/1 -> Multiply5/1
  Delay6/1 -> Add3/2
  Rate Transition/1 -> Multiply3/2, Delay5/1

== system final_heart_sym3_2_Level_hdl/Subsystem/1st_Level_Recon/HiR_Even ==
  In_HiR_e : Inport  OutDataTypeStr=fixdt(1,16,4)  SampleTime=1/44100
  Add : Sum  AccumDataTypeStr=fixdt(1,16,4)  OutDataTypeStr=fixdt(1,16,4)
  Add1 : Sum  AccumDataTypeStr=fixdt(1,16,4)  OutDataTypeStr=fixdt(1,16,4)
  Delay{,1..3} (4 alike) : Delay  DelayLength=1  SampleTime=1/44100
  HiR_0 : Constant  Value=0.035226292  OutDataTypeStr=fixdt(0,16,20)  SampleTime=1/44100
  HiR_2 : Constant  Value=-0.13501102  OutDataTypeStr=fixdt(1,16,17)  SampleTime=1/44100
  HiR_4 : Constant  Value=0.806891509  OutDataTypeStr=fixdt(0,16,16)  SampleTime=1/44100
  Multiply : Product  OutDataTypeStr=fixdt(1,16,4)
  Multiply1 : Product  OutDataTypeStr=fixdt(1,16,4)
  Multiply2 : Product  OutDataTypeStr=fixdt(1,16,4)
  Rate Transition : RateTransition
  Rate Transition1 : RateTransition
  Out_HiR_e : Outport  OutDataTypeStr=fixdt(1,16,4)  SampleTime=1/44100  VectorParamsAs1DForOutWhenUnconnected=off
  wires:
  Delay3/1 -> Add/2
  In_HiR_e/1 -> Delay/1, Multiply/2
  HiR_4/1 -> Multiply2/1
  Multiply/1 -> Add/1
  Add1/1 -> Delay3/1
  Multiply2/1 -> Delay2/1
  Multiply1/1 -> Add1/1
  Delay2/1 -> Add1/2
  Add/1 -> Out_HiR_e/1
  HiR_0/1 -> Multiply/1
  HiR_2/1 -> Multiply1/1
  Delay1/1 -> Rate Transition1/1
  Rate Transition/1 -> Delay1/1, Multiply1/2
  Rate Transition1/1 -> Multiply2/2
  Delay/1 -> Rate Transition/1

== system final_heart_sym3_2_Level_hdl/Subsystem/1st_Level_Recon/HiR_Odd ==
  In_HiR_o : Inport  OutDataTypeStr=fixdt(1,16,4)  SampleTime=1/44100
  Add : Sum  AccumDataTypeStr=fixdt(1,16,4)  OutDataTypeStr=fixdt(1,16,4)
  Add1 : Sum  AccumDataTypeStr=fixdt(1,16,4)  OutDataTypeStr=fixdt(1,16,4)
  Delay{,1..3} (4 alike) : Delay  DelayLength=1  SampleTime=1/44100
  HiR_1 : Constant  Value=0.085441274  OutDataTypeStr=fixdt(0,16,19)  SampleTime=1/44100
  HiR_3 : Constant  Value=-0.459877502  OutDataTypeStr=fixdt(1,16,16)  SampleTime=1/44100
  HiR_5 : Constant  Value=-0.332670553  OutDataTypeStr=fixdt(1,16,16)  SampleTime=1/44100
  Multiply : Product  OutDataTypeStr=fixdt(1,16,4)
  Multiply1 : Product  OutDataTypeStr=fixdt(1,16,4)
  Multiply2 : Product  OutDataTypeStr=fixdt(1,16,4)
  Rate Transition : RateTransition
  Rate Transition1 : RateTransition
  Out_HiR_o : Outport  OutDataTypeStr=fixdt(1,16,4)  SampleTime=1/44100  VectorParamsAs1DForOutWhenUnconnected=off
  wires:
  Delay/1 -> Rate Transition/1
  Rate Transition1/1 -> Multiply2/2
  Delay2/1 -> Add1/2
  HiR_1/1 -> Multiply/1
  Add/1 -> Out_HiR_o/1
  Delay1/1 -> Rate Transition1/1
  HiR_3/1 -> Multiply1/1
  Multiply1/1 -> Add1/1
  Rate Transition/1 -> Delay1/1, Multiply1/2
  Add1/1 -> Delay3/1
  Multiply/1 -> Add/1
  In_HiR_o/1 -> Delay/1, Multiply/2
  Multiply2/1 -> Delay2/1
  HiR_5/1 -> Multiply2/1
  Delay3/1 -> Add/2

== system final_heart_sym3_2_Level_hdl/Subsystem/1st_Level_Recon/LoR_Even ==
  In_LoR_e : Inport  OutDataTypeStr=fixdt(1,16,4)  SampleTime=1/44100
  Add : Sum  AccumDataTypeStr=fixdt(1,16,4)  OutDataTypeStr=fixdt(1,16,4)
  Add1 : Sum  AccumDataTypeStr=fixdt(1,16,4)  OutDataTypeStr=fixdt(1,16,4)
  Delay{,1..3} (4 alike) : Delay  DelayLength=1  SampleTime=1/44100
  LoR_0 : Constant  Value=0.332670553  OutDataTypeStr=fixdt(0,16,17)  SampleTime=1/44100
  LoR_2 : Constant  Value=0.459877502  OutDataTypeStr=fixdt(0,16,17)  SampleTime=1/44100
  LoR_4 : Constant  Value=-0.085441274  OutDataTypeStr=fixdt(1,16,18)  SampleTime=1/44100
  Multiply : Product  OutDataTypeStr=fixdt(1,16,4)
  Multiply1 : Product  OutDataTypeStr=fixdt(1,16,4)
  Multiply2 : Product  OutDataTypeStr=fixdt(1,16,4)
  Rate Transition : RateTransition
  Rate Transition1 : RateTransition
  Out_LoR_e : Outport  OutDataTypeStr=fixdt(1,16,4)  SampleTime=1/44100  VectorParamsAs1DForOutWhenUnconnected=off
  wires:
  Delay/1 -> Rate Transition/1
  Rate Transition1/1 -> Multiply2/2
  Delay2/1 -> Add1/2
  LoR_0/1 -> Multiply/1
  Add/1 -> Out_LoR_e/1
  Delay1/1 -> Rate Transition1/1
  LoR_2/1 -> Multiply1/1
  Multiply1/1 -> Add1/1
  Rate Transition/1 -> Delay1/1, Multiply1/2
  Add1/1 -> Delay3/1
  Multiply/1 -> Add/1
  In_LoR_e/1 -> Delay/1, Multiply/2
  Multiply2/1 -> Delay2/1
  LoR_4/1 -> Multiply2/1
  Delay3/1 -> Add/2

== system final_heart_sym3_2_Level_hdl/Subsystem/1st_Level_Recon/LoR_Odd ==
  In_LoR_o : Inport  OutDataTypeStr=fixdt(1,16,4)  SampleTime=1/44100
  Add : Sum  AccumDataTypeStr=fixdt(1,16,4)  OutDataTypeStr=fixdt(1,16,4)
  Add1 : Sum  AccumDataTypeStr=fixdt(1,16,4)  OutDataTypeStr=fixdt(1,16,4)
  Delay{,1..3} (4 alike) : Delay  DelayLength=1  SampleTime=1/44100
  LoR_1 : Constant  Value=0.806891509  OutDataTypeStr=fixdt(0,16,16)  SampleTime=1/44100
  LoR_3 : Constant  Value=-0.13501102  OutDataTypeStr=fixdt(1,16,17)  SampleTime=1/44100
  LoR_5 : Constant  Value=0.035226292  OutDataTypeStr=fixdt(0,16,20)  SampleTime=1/44100
  Multiply : Product  OutDataTypeStr=fixdt(1,16,4)
  Multiply1 : Product  OutDataTypeStr=fixdt(1,16,4)
  Multiply2 : Product  OutDataTypeStr=fixdt(1,16,4)
  Rate Transition : RateTransition
  Rate Transition1 : RateTransition
  Out_LoR_o : Outport  OutDataTypeStr=fixdt(1,16,4)  SampleTime=1/44100  VectorParamsAs1DForOutWhenUnconnected=off
  wires:
  Delay/1 -> Rate Transition/1
  Rate Transition1/1 -> Multiply2/2
  Delay2/1 -> Add1/2
  LoR_1/1 -> Multiply/1
  Add/1 -> Out_LoR_o/1
  Delay1/1 -> Rate Transition1/1
  LoR_3/1 -> Multiply1/1
  Multiply1/1 -> Add1/1
  Rate Transition/1 -> Delay1/1, Multiply1/2
  Add1/1 -> Delay3/1
  Multiply/1 -> Add/1
  In_LoR_o/1 -> Delay/1, Multiply/2
  Multiply2/1 -> Delay2/1
  LoR_5/1 -> Multiply2/1
  Delay3/1 -> Add/2

== system final_heart_sym3_2_Level_hdl/Subsystem/1st_Level_Recon1/HiR_Even ==
  In_HiR_e : Inport  OutDataTypeStr=fixdt(1,16,28)  SampleTime=1/44100
  Add : Sum  AccumDataTypeStr=fixdt(1,16,28)  OutDataTypeStr=fixdt(1,16,28)
  Add1 : Sum  AccumDataTypeStr=fixdt(1,16,28)  OutDataTypeStr=fixdt(1,16,28)
  Delay{,1..3} (4 alike) : Delay  DelayLength=1  SampleTime=1/44100
  HiR_0 : Constant  Value=0.035226292  OutDataTypeStr=fixdt(0,16,20)  SampleTime=1/44100
  HiR_2 : Constant  Value=-0.13501102  OutDataTypeStr=fixdt(1,16,17)  SampleTime=1/44100
  HiR_4 : Constant  Value=0.806891509  OutDataTypeStr=fixdt(0,16,16)  SampleTime=1/44100
  Multiply : Product  OutDataTypeStr=fixdt(1,16,33)
  Multiply1 : Product  OutDataTypeStr=fixdt(1,16,31)
  Multiply2 : Product  OutDataTypeStr=fixdt(1,16,28)
  Rate Transition : RateTransition
  Rate Transition1 : RateTransition
  Out_HiR_e : Outport  OutDataTypeStr=fixdt(1,16,28)  SampleTime=1/44100  VectorParamsAs1DForOutWhenUnconnected=off
  wires:
  Delay3/1 -> Add/2
  In_HiR_e/1 -> Delay/1, Multiply/2
  HiR_4/1 -> Multiply2/1
  Multiply/1 -> Add/1
  Add1/1 -> Delay3/1
  Multiply2/1 -> Delay2/1
  Multiply1/1 -> Add1/1
  Delay2/1 -> Add1/2
  Add/1 -> Out_HiR_e/1
  HiR_0/1 -> Multiply/1
  HiR_2/1 -> Multiply1/1
  Delay1/1 -> Rate Transition1/1
  Rate Transition/1 -> Delay1/1, Multiply1/2
  Rate Transition1/1 -> Multiply2/2
  Delay/1 -> Rate Transition/1

== system final_heart_sym3_2_Level_hdl/Subsystem/1st_Level_Recon1/HiR_Odd ==
  In_HiR_o : Inport  OutDataTypeStr=fixdt(1,16,28)  SampleTime=1/44100
  Add : Sum  AccumDataTypeStr=fixdt(1,16,28)  OutDataTypeStr=fixdt(1,16,28)
  Add1 : Sum  AccumDataTypeStr=fixdt(1,16,28)  OutDataTypeStr=fixdt(1,16,28)
  Delay{,1..3} (4 alike) : Delay  DelayLength=1  SampleTime=1/44100
  HiR_1 : Constant  Value=0.085441274  OutDataTypeStr=fixdt(0,16,19)  SampleTime=1/44100
  HiR_3 : Constant  Value=-0.459877502  OutDataTypeStr=fixdt(1,16,16)  SampleTime=1/44100
  HiR_5 : Constant  Value=-0.332670553  OutDataTypeStr=fixdt(1,16,16)  SampleTime=1/44100
  Multiply : Product  OutDataTypeStr=fixdt(1,16,31)
  Multiply1 : Product  OutDataTypeStr=fixdt(1,16,29)
  Multiply2 : Product  OutDataTypeStr=fixdt(1,16,29)
  Rate Transition : RateTransition
  Rate Transition1 : RateTransition
  Out_HiR_o : Outport  OutDataTypeStr=fixdt(1,16,28)  SampleTime=1/44100  VectorParamsAs1DForOutWhenUnconnected=off
  wires:
  Delay/1 -> Rate Transition/1
  Rate Transition1/1 -> Multiply2/2
  Delay2/1 -> Add1/2
  HiR_1/1 -> Multiply/1
  Add/1 -> Out_HiR_o/1
  Delay1/1 -> Rate Transition1/1
  HiR_3/1 -> Multiply1/1
  Multiply1/1 -> Add1/1
  Rate Transition/1 -> Delay1/1, Multiply1/2
  Add1/1 -> Delay3/1
  Multiply/1 -> Add/1
  In_HiR_o/1 -> Delay/1, Multiply/2
  Multiply2/1 -> Delay2/1
  HiR_5/1 -> Multiply2/1
  Delay3/1 -> Add/2

== system final_heart_sym3_2_Level_hdl/Subsystem/1st_Level_Recon1/LoR_Even ==
  In_LoR_e : Inport  OutDataTypeStr=fixdt(1,16,4)  SampleTime=1/44100
  Add : Sum  AccumDataTypeStr=fixdt(1,16,4)  OutDataTypeStr=fixdt(1,16,4)
  Add1 : Sum  AccumDataTypeStr=fixdt(1,16,4)  OutDataTypeStr=fixdt(1,16,4)
  Delay{,1..3} (4 alike) : Delay  DelayLength=1  SampleTime=1/44100
  LoR_0 : Constant  Value=0.332670553  OutDataTypeStr=fixdt(0,16,17)  SampleTime=1/44100
  LoR_2 : Constant  Value=0.459877502  OutDataTypeStr=fixdt(0,16,17)  SampleTime=1/44100
  LoR_4 : Constant  Value=-0.085441274  OutDataTypeStr=fixdt(1,16,18)  SampleTime=1/44100
  Multiply : Product  OutDataTypeStr=fixdt(1,16,4)
  Multiply1 : Product  OutDataTypeStr=fixdt(1,16,4)
  Multiply2 : Product  OutDataTypeStr=fixdt(1,16,4)
  Rate Transition : RateTransition
  Rate Transition1 : RateTransition
  Out_LoR_e : Outport  OutDataTypeStr=fixdt(1,16,4)  SampleTime=1/44100  VectorParamsAs1DForOutWhenUnconnected=off
  wires:
  Delay/1 -> Rate Transition/1
  Rate Transition1/1 -> Multiply2/2
  Delay2/1 -> Add1/2
  LoR_0/1 -> Multiply/1
  Add/1 -> Out_LoR_e/1
  Delay1/1 -> Rate Transition1/1
  LoR_2/1 -> Multiply1/1
  Multiply1/1 -> Add1/1
  Rate Transition/1 -> Delay1/1, Multiply1/2
  Add1/1 -> Delay3/1
  Multiply/1 -> Add/1
  In_LoR_e/1 -> Delay/1, Multiply/2
  Multiply2/1 -> Delay2/1
  LoR_4/1 -> Multiply2/1
  Delay3/1 -> Add/2

== system final_heart_sym3_2_Level_hdl/Subsystem/1st_Level_Recon1/LoR_Odd ==
  In_LoR_o : Inport  OutDataTypeStr=fixdt(1,16,4)  SampleTime=1/44100
  Add : Sum  AccumDataTypeStr=fixdt(1,16,4)  OutDataTypeStr=fixdt(1,16,4)
  Add1 : Sum  AccumDataTypeStr=fixdt(1,16,4)  OutDataTypeStr=fixdt(1,16,4)
  Delay{,1..3} (4 alike) : Delay  DelayLength=1  SampleTime=1/44100
  LoR_1 : Constant  Value=0.806891509  OutDataTypeStr=fixdt(0,16,16)  SampleTime=1/44100
  LoR_3 : Constant  Value=-0.13501102  OutDataTypeStr=fixdt(1,16,17)  SampleTime=1/44100
  LoR_5 : Constant  Value=0.035226292  OutDataTypeStr=fixdt(0,16,20)  SampleTime=1/44100
  Multiply : Product  OutDataTypeStr=fixdt(1,16,4)
  Multiply1 : Product  OutDataTypeStr=fixdt(1,16,4)
  Multiply2 : Product  OutDataTypeStr=fixdt(1,16,4)
  Rate Transition : RateTransition
  Rate Transition1 : RateTransition
  Out_LoR_o : Outport  OutDataTypeStr=fixdt(1,16,4)  SampleTime=1/44100  VectorParamsAs1DForOutWhenUnconnected=off
  wires:
  Delay/1 -> Rate Transition/1
  Rate Transition1/1 -> Multiply2/2
  Delay2/1 -> Add1/2
  LoR_1/1 -> Multiply/1
  Add/1 -> Out_LoR_o/1
  Delay1/1 -> Rate Transition1/1
  LoR_3/1 -> Multiply1/1
  Multiply1/1 -> Add1/1
  Rate Transition/1 -> Delay1/1, Multiply1/2
  Add1/1 -> Delay3/1
  Multiply/1 -> Add/1
  In_LoR_o/1 -> Delay/1, Multiply/2
  Multiply2/1 -> Delay2/1
  LoR_5/1 -> Multiply2/1
  Delay3/1 -> Add/2

== system final_heart_sym3_2_Level_hdl/Subsystem/Threshold_Estimator/Absolute_Value1 ==
  Signal_w4 : Inport  OutDataTypeStr=fixdt(1,16,4)  SampleTime=1/44100
  Absolute_Switch : Switch  Threshold=1  OutDataTypeStr=fixdt(1,16,4)
  Constant295 : Constant  Value=0  OutDataTypeStr=fixdt(1,16,4)  SampleTime=1/44100
  Gain2 : Gain  Gain=-1  ParamDataTypeStr=fixdt(1,16,15)  OutDataTypeStr=fixdt(1,16,4)
  Relational Operator2 : RelationalOperator  Operator=<  OutDataTypeStr=boolean  RndMeth=Simplest
  Out_Abs : Outport  OutDataTypeStr=fixdt(1,16,4)  SampleTime=1/44100  VectorParamsAs1DForOutWhenUnconnected=off
  wires:
  Absolute_Switch/1 -> Out_Abs/1
  Relational Operator2/1 -> Absolute_Switch/2
  Gain2/1 -> Absolute_Switch/1
  Signal_w4/1 -> Absolute_Switch/3, Relational Operator2/1, Gain2/1
  Constant295/1 -> Relational Operator2/2

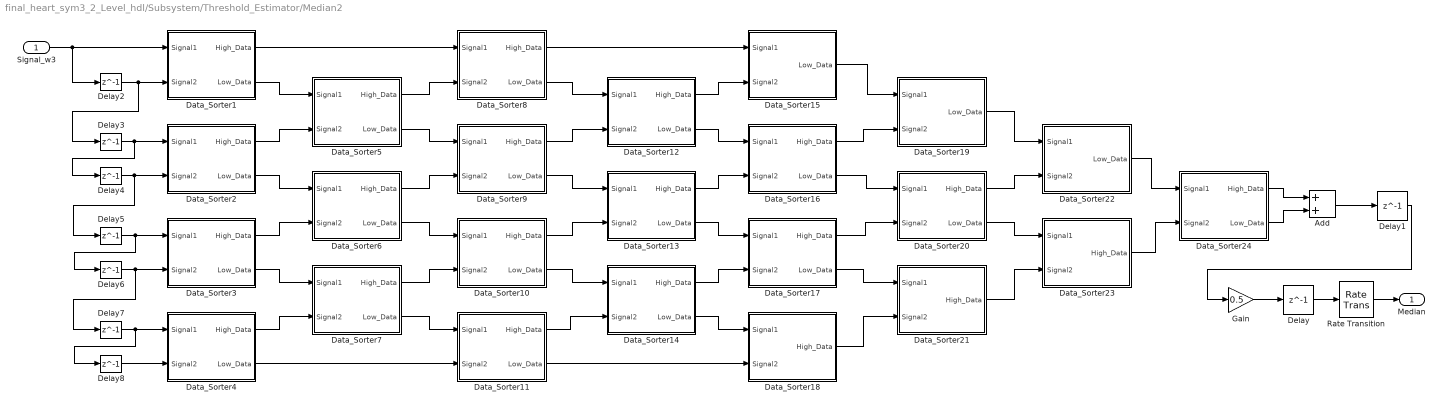
== system final_heart_sym3_2_Level_hdl/Subsystem/Threshold_Estimator/Median2 ==
  Signal_w3 : Inport  OutDataTypeStr=fixdt(1,16,4)  SampleTime=1/44100
  Add : Sum  AccumDataTypeStr=fixdt(1,16,4)  OutDataTypeStr=fixdt(1,16,4)
  Data_Sorter1 : Subsystem
  Data_Sorter10 : Subsystem
  Data_Sorter11 : Subsystem
  Data_Sorter12 : Subsystem
  Data_Sorter13 : Subsystem
  Data_Sorter14 : Subsystem
  Data_Sorter15 : Subsystem
  Data_Sorter16 : Subsystem
  Data_Sorter17 : Subsystem
  Data_Sorter18 : Subsystem
  Data_Sorter19 : Subsystem
  Data_Sorter2 : Subsystem
  Data_Sorter20 : Subsystem
  Data_Sorter21 : Subsystem
  Data_Sorter22 : Subsystem
  Data_Sorter23 : Subsystem
  Data_Sorter24 : Subsystem
  Data_Sorter3 : Subsystem
  Data_Sorter4 : Subsystem
  Data_Sorter5 : Subsystem
  Data_Sorter6 : Subsystem
  Data_Sorter7 : Subsystem
  Data_Sorter8 : Subsystem
  Data_Sorter9 : Subsystem
  Delay{,1..8} (9 alike) : Delay  DelayLength=1  SampleTime=1/44100
  Gain : Gain  Gain=0.5  ParamDataTypeStr=fixdt(0,16,16)  OutDataTypeStr=fixdt(1,16,4)
  Rate Transition : RateTransition
  Median : Outport  OutDataTypeStr=fixdt(1,16,4)  SampleTime=1/44100  VectorParamsAs1DForOutWhenUnconnected=off
  wires:
  Data_Sorter4/1(High_Data) -> Data_Sorter7/2(Signal2)
  Delay3/1 -> Data_Sorter2/1(Signal1), Delay4/1
  Signal_w3/1 -> Data_Sorter1/1(Signal1), Delay2/1
  Data_Sorter10/1(High_Data) -> Data_Sorter13/2(Signal2)
  Data_Sorter23/1(High_Data) -> Data_Sorter24/2(Signal2)
  Data_Sorter12/2(Low_Data) -> Data_Sorter16/1(Signal1)
  Delay2/1 -> Delay3/1, Data_Sorter1/2(Signal2)
  Data_Sorter5/1(High_Data) -> Data_Sorter8/2(Signal2)
  Delay/1 -> Rate Transition/1
  Data_Sorter15/1(Low_Data) -> Data_Sorter19/1(Signal1)
  Add/1 -> Delay1/1
  Data_Sorter7/2(Low_Data) -> Data_Sorter11/1(Signal1)
  Data_Sorter24/1(High_Data) -> Add/1
  Data_Sorter1/2(Low_Data) -> Data_Sorter5/1(Signal1)
  Data_Sorter3/1(High_Data) -> Data_Sorter6/2(Signal2)
  Data_Sorter22/1(Low_Data) -> Data_Sorter24/1(Signal1)
  Data_Sorter2/1(High_Data) -> Data_Sorter5/2(Signal2)
  Data_Sorter10/2(Low_Data) -> Data_Sorter14/1(Signal1)
  Delay1/1 -> Gain/1
  Data_Sorter17/2(Low_Data) -> Data_Sorter21/1(Signal1)
  Data_Sorter21/1(High_Data) -> Data_Sorter23/2(Signal2)
  Data_Sorter7/1(High_Data) -> Data_Sorter10/2(Signal2)
  Delay4/1 -> Data_Sorter2/2(Signal2), Delay5/1
  Data_Sorter16/1(High_Data) -> Data_Sorter19/2(Signal2)
  Data_Sorter20/1(High_Data) -> Data_Sorter22/2(Signal2)
  Data_Sorter16/2(Low_Data) -> Data_Sorter20/1(Signal1)
  Data_Sorter3/2(Low_Data) -> Data_Sorter7/1(Signal1)
  Data_Sorter2/2(Low_Data) -> Data_Sorter6/1(Signal1)
  Data_Sorter6/2(Low_Data) -> Data_Sorter10/1(Signal1)
  Data_Sorter19/1(Low_Data) -> Data_Sorter22/1(Signal1)
  Data_Sorter12/1(High_Data) -> Data_Sorter15/2(Signal2)
  Data_Sorter5/2(Low_Data) -> Data_Sorter9/1(Signal1)
  Data_Sorter24/2(Low_Data) -> Add/2
  Data_Sorter17/1(High_Data) -> Data_Sorter20/2(Signal2)
  Data_Sorter13/1(High_Data) -> Data_Sorter16/2(Signal2)
  Data_Sorter11/1(High_Data) -> Data_Sorter14/2(Signal2)
  Delay8/1 -> Data_Sorter4/2(Signal2)
  Data_Sorter8/2(Low_Data) -> Data_Sorter12/1(Signal1)
  Delay6/1 -> Data_Sorter3/2(Signal2), Delay7/1
  Data_Sorter9/2(Low_Data) -> Data_Sorter13/1(Signal1)
  Data_Sorter4/2(Low_Data) -> Data_Sorter11/2(Signal2)
  Data_Sorter9/1(High_Data) -> Data_Sorter12/2(Signal2)
  Data_Sorter14/2(Low_Data) -> Data_Sorter18/1(Signal1)
  Delay5/1 -> Data_Sorter3/1(Signal1), Delay6/1
  Delay7/1 -> Data_Sorter4/1(Signal1), Delay8/1
  Data_Sorter1/1(High_Data) -> Data_Sorter8/1(Signal1)
  Data_Sorter8/1(High_Data) -> Data_Sorter15/1(Signal1)
  Data_Sorter14/1(High_Data) -> Data_Sorter17/2(Signal2)
  Data_Sorter6/1(High_Data) -> Data_Sorter9/2(Signal2)
  Data_Sorter20/2(Low_Data) -> Data_Sorter23/1(Signal1)
  Data_Sorter11/2(Low_Data) -> Data_Sorter18/2(Signal2)
  Data_Sorter13/2(Low_Data) -> Data_Sorter17/1(Signal1)
  Gain/1 -> Delay/1
  Data_Sorter18/1(High_Data) -> Data_Sorter21/2(Signal2)
  Rate Transition/1 -> Median/1

== system final_heart_sym3_2_Level_hdl/Subsystem/Threshold_Estimator/Median2/Data_Sorter1 ==
  Signal1 : Inport  OutDataTypeStr=fixdt(1,16,4)  SampleTime=1/44100
  Signal2 : Inport  Port=2  OutDataTypeStr=fixdt(1,16,4)  SampleTime=1/44100
  Data_Sorter_Switch : Switch  OutDataTypeStr=fixdt(1,16,4)
  Data_Sorter_Switch1 : Switch  Threshold=1  OutDataTypeStr=fixdt(1,16,4)
  Delay1 : Delay  DelayLength=1  SampleTime=1/44100
  Delay2 : Delay  DelayLength=1  SampleTime=1/44100
  Relational Operator2 : RelationalOperator  Operator=<  OutDataTypeStr=boolean  RndMeth=Simplest
  High_Data : Outport  OutDataTypeStr=fixdt(1,16,4)  SampleTime=1/44100  VectorParamsAs1DForOutWhenUnconnected=off
  Low_Data : Outport  Port=2  OutDataTypeStr=fixdt(1,16,4)  SampleTime=1/44100  VectorParamsAs1DForOutWhenUnconnected=off
  wires:
  Signal1/1 -> Data_Sorter_Switch/3, Data_Sorter_Switch/1, Relational Operator2/1
  Relational Operator2/1 -> Data_Sorter_Switch1/2, Data_Sorter_Switch/2
  Signal2/1 -> Data_Sorter_Switch1/1, Data_Sorter_Switch1/3, Relational Operator2/2
  Data_Sorter_Switch1/1 -> Delay2/1
  Delay2/1 -> Low_Data/1
  Data_Sorter_Switch/1 -> Delay1/1
  Delay1/1 -> High_Data/1

== system final_heart_sym3_2_Level_hdl/Subsystem/Threshold_Estimator/Median2/Data_Sorter10 ==
  Signal1 : Inport  OutDataTypeStr=fixdt(1,16,4)  SampleTime=1/44100
  Signal2 : Inport  Port=2  OutDataTypeStr=fixdt(1,16,4)  SampleTime=1/44100
  Data_Sorter_Switch : Switch  OutDataTypeStr=fixdt(1,16,4)
  Data_Sorter_Switch1 : Switch  Threshold=1  OutDataTypeStr=fixdt(1,16,4)
  Delay1 : Delay  DelayLength=1  SampleTime=1/44100
  Delay2 : Delay  DelayLength=1  SampleTime=1/44100
  Relational Operator2 : RelationalOperator  Operator=<  OutDataTypeStr=boolean  RndMeth=Simplest
  High_Data : Outport  OutDataTypeStr=fixdt(1,16,4)  SampleTime=1/44100  VectorParamsAs1DForOutWhenUnconnected=off
  Low_Data : Outport  Port=2  OutDataTypeStr=fixdt(1,16,4)  SampleTime=1/44100  VectorParamsAs1DForOutWhenUnconnected=off
  wires:
  Signal1/1 -> Data_Sorter_Switch/3, Data_Sorter_Switch/1, Relational Operator2/1
  Relational Operator2/1 -> Data_Sorter_Switch1/2, Data_Sorter_Switch/2
  Signal2/1 -> Data_Sorter_Switch1/1, Data_Sorter_Switch1/3, Relational Operator2/2
  Data_Sorter_Switch1/1 -> Delay2/1
  Delay2/1 -> Low_Data/1
  Data_Sorter_Switch/1 -> Delay1/1
  Delay1/1 -> High_Data/1

== system final_heart_sym3_2_Level_hdl/Subsystem/Threshold_Estimator/Median2/Data_Sorter11 ==
  Signal1 : Inport  OutDataTypeStr=fixdt(1,16,4)  SampleTime=1/44100
  Signal2 : Inport  Port=2  OutDataTypeStr=fixdt(1,16,4)  SampleTime=1/44100
  Data_Sorter_Switch : Switch  OutDataTypeStr=fixdt(1,16,4)
  Data_Sorter_Switch1 : Switch  Threshold=1  OutDataTypeStr=fixdt(1,16,4)
  Delay1 : Delay  DelayLength=1  SampleTime=1/44100
  Delay2 : Delay  DelayLength=1  SampleTime=1/44100
  Relational Operator2 : RelationalOperator  Operator=<  OutDataTypeStr=boolean  RndMeth=Simplest
  High_Data : Outport  OutDataTypeStr=fixdt(1,16,4)  SampleTime=1/44100  VectorParamsAs1DForOutWhenUnconnected=off
  Low_Data : Outport  Port=2  OutDataTypeStr=fixdt(1,16,4)  SampleTime=1/44100  VectorParamsAs1DForOutWhenUnconnected=off
  wires:
  Signal1/1 -> Data_Sorter_Switch/3, Data_Sorter_Switch/1, Relational Operator2/1
  Relational Operator2/1 -> Data_Sorter_Switch1/2, Data_Sorter_Switch/2
  Signal2/1 -> Data_Sorter_Switch1/1, Data_Sorter_Switch1/3, Relational Operator2/2
  Data_Sorter_Switch1/1 -> Delay2/1
  Delay2/1 -> Low_Data/1
  Data_Sorter_Switch/1 -> Delay1/1
  Delay1/1 -> High_Data/1

== system final_heart_sym3_2_Level_hdl/Subsystem/Threshold_Estimator/Median2/Data_Sorter12 ==
  Signal1 : Inport  OutDataTypeStr=fixdt(1,16,4)  SampleTime=1/44100
  Signal2 : Inport  Port=2  OutDataTypeStr=fixdt(1,16,4)  SampleTime=1/44100
  Data_Sorter_Switch : Switch  OutDataTypeStr=fixdt(1,16,4)
  Data_Sorter_Switch1 : Switch  Threshold=1  OutDataTypeStr=fixdt(1,16,4)
  Delay1 : Delay  DelayLength=1  SampleTime=1/44100
  Delay2 : Delay  DelayLength=1  SampleTime=1/44100
  Relational Operator2 : RelationalOperator  Operator=<  OutDataTypeStr=boolean  RndMeth=Simplest
  High_Data : Outport  OutDataTypeStr=fixdt(1,16,4)  SampleTime=1/44100  VectorParamsAs1DForOutWhenUnconnected=off
  Low_Data : Outport  Port=2  OutDataTypeStr=fixdt(1,16,4)  SampleTime=1/44100  VectorParamsAs1DForOutWhenUnconnected=off
  wires:
  Signal1/1 -> Data_Sorter_Switch/3, Data_Sorter_Switch/1, Relational Operator2/1
  Relational Operator2/1 -> Data_Sorter_Switch1/2, Data_Sorter_Switch/2
  Signal2/1 -> Data_Sorter_Switch1/1, Data_Sorter_Switch1/3, Relational Operator2/2
  Data_Sorter_Switch1/1 -> Delay2/1
  Delay2/1 -> Low_Data/1
  Data_Sorter_Switch/1 -> Delay1/1
  Delay1/1 -> High_Data/1

== system final_heart_sym3_2_Level_hdl/Subsystem/Threshold_Estimator/Median2/Data_Sorter13 ==
  Signal1 : Inport  OutDataTypeStr=fixdt(1,16,4)  SampleTime=1/44100
  Signal2 : Inport  Port=2  OutDataTypeStr=fixdt(1,16,4)  SampleTime=1/44100
  Data_Sorter_Switch : Switch  OutDataTypeStr=fixdt(1,16,4)
  Data_Sorter_Switch1 : Switch  Threshold=1  OutDataTypeStr=fixdt(1,16,4)
  Delay1 : Delay  DelayLength=1  SampleTime=1/44100
  Delay2 : Delay  DelayLength=1  SampleTime=1/44100
  Relational Operator2 : RelationalOperator  Operator=<  OutDataTypeStr=boolean  RndMeth=Simplest
  High_Data : Outport  OutDataTypeStr=fixdt(1,16,4)  SampleTime=1/44100  VectorParamsAs1DForOutWhenUnconnected=off
  Low_Data : Outport  Port=2  OutDataTypeStr=fixdt(1,16,4)  SampleTime=1/44100  VectorParamsAs1DForOutWhenUnconnected=off
  wires:
  Signal1/1 -> Data_Sorter_Switch/3, Data_Sorter_Switch/1, Relational Operator2/1
  Relational Operator2/1 -> Data_Sorter_Switch1/2, Data_Sorter_Switch/2
  Signal2/1 -> Data_Sorter_Switch1/1, Data_Sorter_Switch1/3, Relational Operator2/2
  Data_Sorter_Switch1/1 -> Delay2/1
  Delay2/1 -> Low_Data/1
  Data_Sorter_Switch/1 -> Delay1/1
  Delay1/1 -> High_Data/1

== system final_heart_sym3_2_Level_hdl/Subsystem/Threshold_Estimator/Median2/Data_Sorter14 ==
  Signal1 : Inport  OutDataTypeStr=fixdt(1,16,4)  SampleTime=1/44100
  Signal2 : Inport  Port=2  OutDataTypeStr=fixdt(1,16,4)  SampleTime=1/44100
  Data_Sorter_Switch : Switch  OutDataTypeStr=fixdt(1,16,4)
  Data_Sorter_Switch1 : Switch  Threshold=1  OutDataTypeStr=fixdt(1,16,4)
  Delay1 : Delay  DelayLength=1  SampleTime=1/44100
  Delay2 : Delay  DelayLength=1  SampleTime=1/44100
  Relational Operator2 : RelationalOperator  Operator=<  OutDataTypeStr=boolean  RndMeth=Simplest
  High_Data : Outport  OutDataTypeStr=fixdt(1,16,4)  SampleTime=1/44100  VectorParamsAs1DForOutWhenUnconnected=off
  Low_Data : Outport  Port=2  OutDataTypeStr=fixdt(1,16,4)  SampleTime=1/44100  VectorParamsAs1DForOutWhenUnconnected=off
  wires:
  Signal1/1 -> Data_Sorter_Switch/3, Data_Sorter_Switch/1, Relational Operator2/1
  Relational Operator2/1 -> Data_Sorter_Switch1/2, Data_Sorter_Switch/2
  Signal2/1 -> Data_Sorter_Switch1/1, Data_Sorter_Switch1/3, Relational Operator2/2
  Data_Sorter_Switch1/1 -> Delay2/1
  Delay2/1 -> Low_Data/1
  Data_Sorter_Switch/1 -> Delay1/1
  Delay1/1 -> High_Data/1
